simulink model "Trac_Energy_Analysis"  (R2018a)
settings: Solver=VariableStepAuto  StartTime=0.0  StopTime=1220  RelTol=1e-3
libraries: qss_tb_library x2, simulink x1
settings Model: Creator=egp  LastModifiedBy=egp

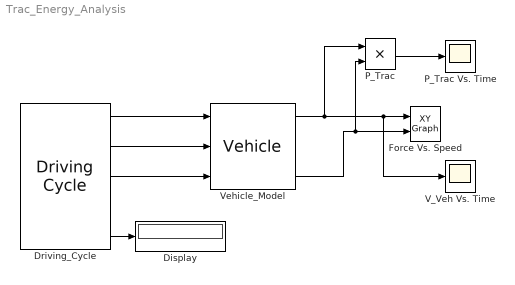
== system Trac_Energy_Analysis ==
  Display : Display
  Driving_Cycle : qss_tb_library/Driving Cycle/Driving Cycle  Tag=cycle  cyclename1=NEDC  stepsize=1  autostop=on
  Force Vs. Speed : simulink/Sinks/XY Graph  xmin=0  xmax=40  ymin=-2500  ymax=2500  st=-1
  P_Trac : Product
  P_Trac Vs. Time : Scope
  V_Veh Vs. Time : Scope
  Vehicle_Model : qss_tb_library/Vehicle/Vehicle  Tag=vehicle  m_f=1750  A_f=2.88  cw=0.5  mu=0.01  k_inertia=5
  wires:
  Driving_Cycle/1 -> Vehicle_Model/1
  Driving_Cycle/2 -> Vehicle_Model/2
  Driving_Cycle/3 -> Vehicle_Model/3
  Vehicle_Model/1 -> P_Trac/1, V_Veh Vs. Time/1, Force Vs. Speed/1
  Vehicle_Model/3 -> P_Trac/2, Force Vs. Speed/2
  P_Trac/1 -> P_Trac Vs. Time/1
  Driving_Cycle/5 -> Display/1
